simulink model "Pendulum"  (R2023a)
settings: Solver=ode45  StartTime=0.0  StopTime=10  RelTol=1e-3
model workspace (MAT data in the model file):
  A = 0.01
  b = 50
  k = 50
  m = 250
  omega = 1
values from neighbouring files (symbols this model uses):
  g = 9.81    [constants.m]
  J = 1.9098e-4    (= 0.00019098)    [constants.m]
  K = 53.6e-3    (= 0.0536)    [constants.m]
  Km = K/R    (= 0.00564210526316)    [constants.m]
  l = 0.042    [constants.m]
  R = 1    [constants.m]
settings Model: VariantFading=off  Creator=Researcher  LastModifiedBy=qnmdgpqs

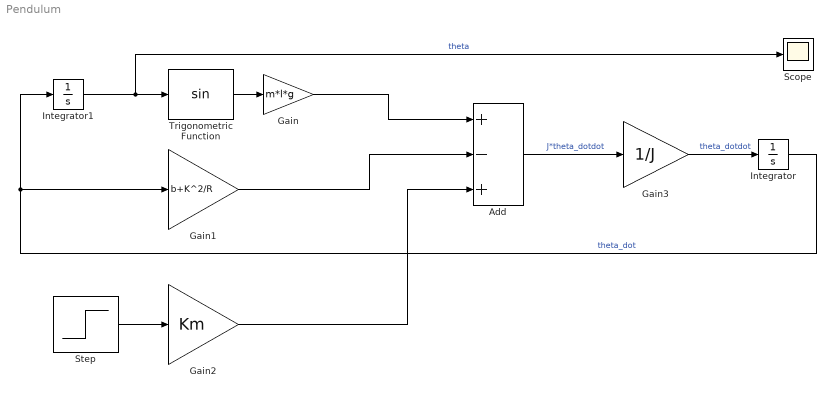
== system Pendulum ==
  Add : Sum  Inputs=+-+
  Gain : Gain  Gain=m*l*g
  Gain1 : Gain  Gain=b+K^2/R
  Gain2 : Gain  Gain=Km
  Gain3 : Gain  Gain=1/J
  Integrator : Integrator
  Integrator1 : Integrator  InitialCondition=pi
  Scope : Scope
  Step : Step  SampleTime=0
  Trigonometric Function : Trigonometry
  wires:
  Integrator1/1 -> Scope/1, Trigonometric Function/1  "theta"
  Trigonometric Function/1 -> Gain/1
  Gain/1 -> Add/1
  Integrator/1 -> Gain1/1, Integrator1/1  "theta_dot"
  Gain1/1 -> Add/2
  Step/1 -> Gain2/1
  Gain2/1 -> Add/3
  Add/1 -> Gain3/1  "J*theta_dotdot"
  Gain3/1 -> Integrator/1  "theta_dotdot"
